simulink model "miniprojekt_transmitancja"  (R2020a)
settings: Solver=VariableStepAuto  StartTime=0.0  StopTime=10.0  RelTol=1e-3
values from neighbouring files (symbols this model uses):
  d_qg = 0    [nieliniowy.m]    (also in nieliniowy_leveled.m; statespace_transmitancja.m; statespace_transmitancja_leveled.m)
  d_Tzew = 2    [nieliniowy.m]    (also in nieliniowy_leveled.m; statespace_transmitancja.m; statespace_transmitancja_leveled.m)
  Tp0 = (c_p*ro_p*fp1*qg1)/(c_p*ro_p*fp1*(Kp+Kw)+Kw*Kp)+Tzew1    (= 13.9051724138)    [nieliniowy.m]    (also in nieliniowy_leveled.m; statespace_transmitancja.m = 14.0480349345; statespace_transmitancja_leveled.m = 14.0770577933)
  Twew0 = (c_p*ro_p*fp1*Tp0+Kp*Tp0-Kp*Tzew1)/(c_p*ro_p*fp1)    (= 14.8965517241)    [nieliniowy.m]    (also in nieliniowy_leveled.m; statespace_transmitancja.m = 14.2991266376; statespace_transmitancja_leveled.m = 14.1777583187)
undefined symbols (not defined in the file or in its folder): L1, L2, M1, M2
settings Model: Creator=Jakub Szymkowiak  LastModifiedBy=Jakub Szymkowiak

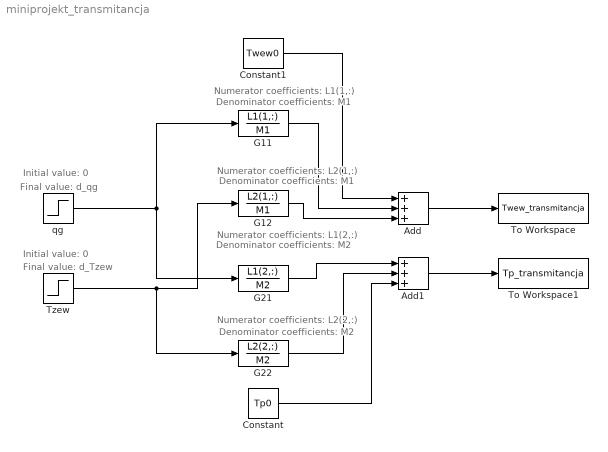
== system miniprojekt_transmitancja ==
  note: Denominator coefficients: M2
  note: Numerator coefficients: L2(2,:)
  note: Denominator coefficients: M2
  note: Numerator coefficients: L1(2,:)
  note: Denominator coefficients: M1
  note: Numerator coefficients: L2(1,:)
  note: Denominator coefficients: M1
  note: Numerator coefficients: L1(1,:)
  note: Final value: d_Tzew
  note: Initial value: 0
  note: Final value: d_qg
  note: Initial value: 0
  Add : Sum  Inputs=+++
  Add1 : Sum  Inputs=+++
  Constant : Constant  Value=Tp0
  Constant1 : Constant  Value=Twew0
  G11 : TransferFcn  Numerator=L1(1,:)  Denominator=M1
  G12 : TransferFcn  Numerator=L2(1,:)  Denominator=M1
  G21 : TransferFcn  Numerator=L1(2,:)  Denominator=M2
  G22 : TransferFcn  Numerator=L2(2,:)  Denominator=M2
  To Workspace : ToWorkspace  VariableName=Twew_transmitancja  SaveFormat=Timeseries  SampleTime=-1
  To Workspace1 : ToWorkspace  VariableName=Tp_transmitancja  SaveFormat=Timeseries  SampleTime=-1
  Tzew : Step  After=d_Tzew  SampleTime=0
  qg : Step  After=d_qg  SampleTime=0
  wires:
  qg/1 -> G21/1, G11/1
  Tzew/1 -> G12/1, G22/1
  Constant1/1 -> Add/1
  G11/1 -> Add/2
  G12/1 -> Add/3
  G21/1 -> Add1/1
  G22/1 -> Add1/2
  Constant/1 -> Add1/3
  Add/1 -> To Workspace/1
  Add1/1 -> To Workspace1/1
